simulink model "DAQModule6"  (R2022a)
settings: Solver=VariableStepAuto  StartTime=0.0  StopTime=2  FixedStep=0.001  RelTol=1e-3
settings Model: Creator=eduyilmet001  LastModifiedBy=eduyilmet001

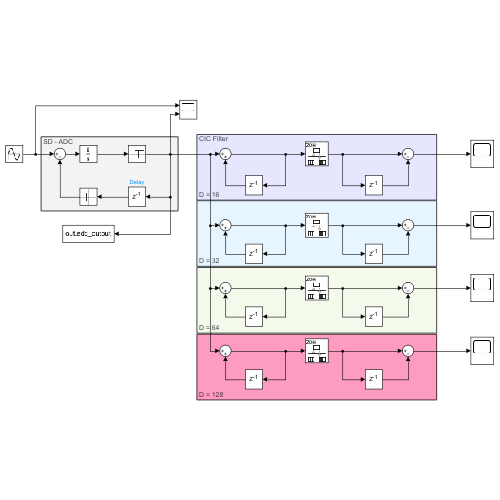
[thumbnail: Simulink's stored preview of the top-level diagram]
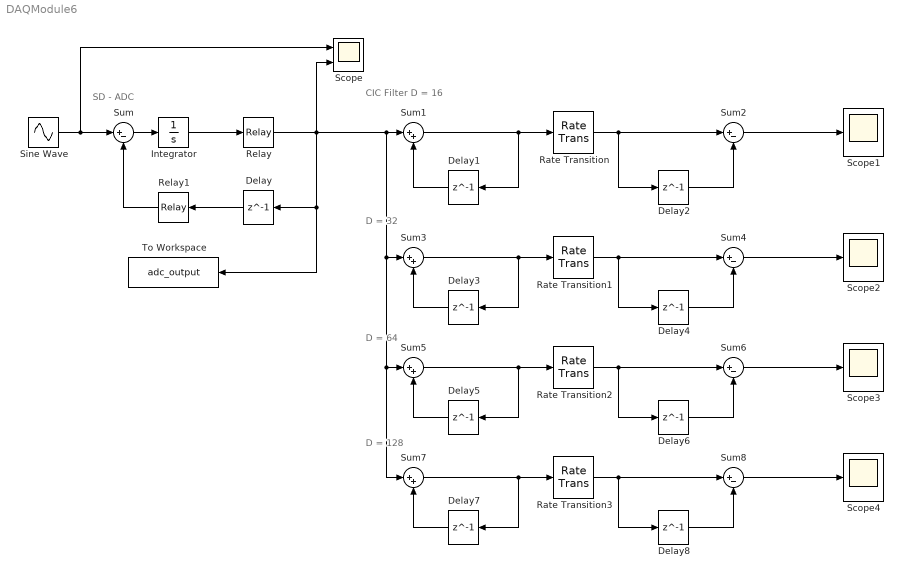
== system DAQModule6 ==
  note: SD - ADC
  note: CIC Filter
      |
      |
      |
      |
      |
      |
      | D = 16
  note: D = 32
  note: D = 64
  note: D = 128
  Delay : Delay  DelayLength=1  SampleTime=10e-5
  Delay1 : Delay  DelayLength=1  SampleTime=16/10e5
  Delay2 : Delay  DelayLength=1  SampleTime=16/10e5
  Delay3 : Delay  DelayLength=1  SampleTime=32/10e5
  Delay4 : Delay  DelayLength=1  SampleTime=32/10e5
  Delay5 : Delay  DelayLength=1  SampleTime=64/10e5
  Delay6 : Delay  DelayLength=1  SampleTime=64/10e5
  Delay7 : Delay  DelayLength=1  SampleTime=128/10e5
  Delay8 : Delay  DelayLength=1  SampleTime=128/10e5
  Integrator : Integrator
  Rate Transition : RateTransition  OutPortSampleTime=16/10e5
  Rate Transition1 : RateTransition  OutPortSampleTime=32/10e5
  Rate Transition2 : RateTransition  OutPortSampleTime=64/10e5
  Rate Transition3 : RateTransition  OutPortSampleTime=128/10e5
  Relay : Relay  OnSwitchValue=0  OffSwitchValue=0  OffOutputValue=-1
  Relay1 : Relay  OnSwitchValue=0  OffSwitchValue=0  OnOutputValue=5  OffOutputValue=-5
  Scope : Scope  NumInputPorts=2
  Scope{1..4} (4 alike) : Scope
  Sine Wave : Sin  Amplitude=2  Frequency=50*2*pi  SampleTime=0
  Sum{,2,4,6,8} (5 alike) : Sum  Inputs=|+-
  Sum{1,3,5,7} (4 alike) : Sum  Inputs=|++
  To Workspace : ToWorkspace  VariableName=adc_output  SaveFormat=Timeseries  SampleTime=-1
  wires:
  Sum/1 -> Integrator/1
  Integrator/1 -> Relay/1
  Delay/1 -> Relay1/1
  Relay1/1 -> Sum/2
  Sine Wave/1 -> Scope/1, Sum/1
  Relay/1 -> Sum3/1, Sum5/1, Sum7/1, Sum1/1, Scope/2, To Workspace/1, Delay/1
  Delay1/1 -> Sum1/2
  Sum1/1 -> Delay1/1, Rate Transition/1
  Rate Transition/1 -> Delay2/1, Sum2/1
  Delay2/1 -> Sum2/2
  Sum2/1 -> Scope1/1
  Sum4/1 -> Scope2/1
  Delay4/1 -> Sum4/2
  Rate Transition1/1 -> Delay4/1, Sum4/1
  Sum3/1 -> Delay3/1, Rate Transition1/1
  Delay3/1 -> Sum3/2
  Delay5/1 -> Sum5/2
  Sum5/1 -> Rate Transition2/1, Delay5/1
  Rate Transition2/1 -> Sum6/1, Delay6/1
  Delay6/1 -> Sum6/2
  Sum6/1 -> Scope3/1
  Sum8/1 -> Scope4/1
  Delay8/1 -> Sum8/2
  Rate Transition3/1 -> Delay8/1, Sum8/1
  Sum7/1 -> Delay7/1, Rate Transition3/1
  Delay7/1 -> Sum7/2
